simulink model "p7"  (R2020a)
settings: Solver=VariableStepAuto  StartTime=0.0  StopTime=10.0  RelTol=1e-3
model workspace (MAT data in the model file):
  A = Simulink.Parameter
  A.Value = 1
  A.DataType = 'auto'
  A.Dimensions = [1 1]
  B = Simulink.Parameter
  B.Value = 2
  B.DataType = 'auto'
  B.Dimensions = [1 1]
  C = Simulink.Parameter
  C.Value = -1
  C.DataType = 'auto'
  C.Dimensions = [1 1]
  D = Simulink.Parameter
  D.Value = 1
  D.DataType = 'auto'
  D.Dimensions = [1 1]
  E = Simulink.Parameter
  E.Value = 1
  E.DataType = 'auto'
  E.Dimensions = [1 1]
  F = Simulink.Parameter
  F.Value = -1
  F.DataType = 'auto'
  F.Dimensions = [1 1]
settings Model: Creator=007  LastModifiedBy=007

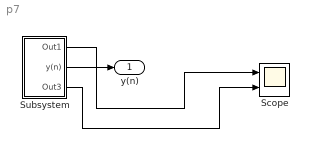
== system p7 ==
  Scope : Scope  NumInputPorts=2
  Subsystem : Subsystem
  y(n) : Outport
  wires:
  Subsystem/1(Out1) -> Scope/1
  Subsystem/2(y(n)) -> y(n)/1
  Subsystem/3(Out3) -> Scope/2

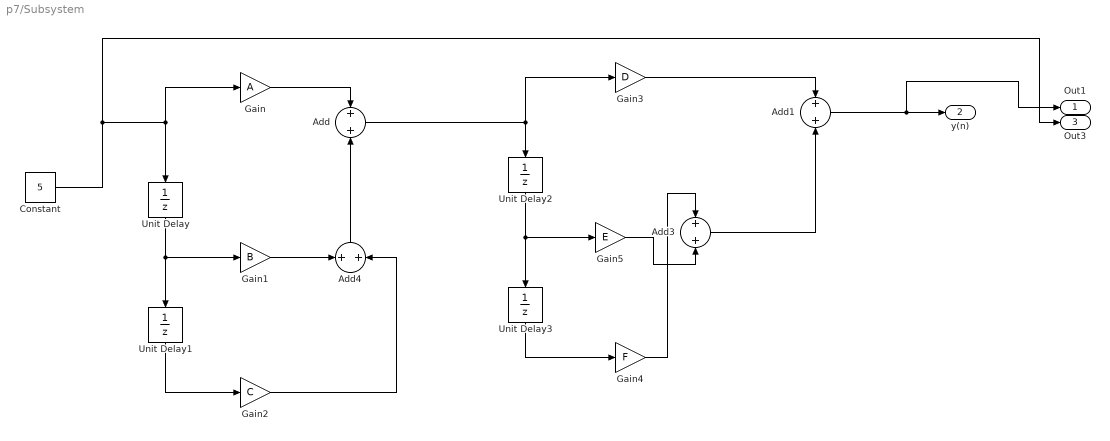
== system p7/Subsystem ==
  Add{,1,3..4} (4 alike) : Sum
  Constant : Constant  Value=5
  Gain : Gain  Gain=A
  Gain1 : Gain  Gain=B
  Gain2 : Gain  Gain=C
  Gain3 : Gain  Gain=D
  Gain4 : Gain  Gain=F
  Gain5 : Gain  Gain=E
  Unit Delay{,1..3} (4 alike) : UnitDelay  SampleTime=-1  HasFrameUpgradeWarning=on
  Out1 : Outport
  y(n) : Outport  Port=2
  Out3 : Outport  Port=3
  wires:
  Add/1 -> Unit Delay2/1, Gain3/1
  Gain/1 -> Add/1
  Gain5/1 -> Add3/2
  Unit Delay2/1 -> Unit Delay3/1, Gain5/1
  Add4/1 -> Add/2
  Add3/1 -> Add1/2
  Unit Delay1/1 -> Gain2/1
  Add1/1 -> y(n)/1, Out1/1
  Gain4/1 -> Add3/1
  Constant/1 -> Out3/1, Unit Delay/1, Gain/1
  Unit Delay3/1 -> Gain4/1
  Unit Delay/1 -> Unit Delay1/1, Gain1/1
  Gain1/1 -> Add4/1
  Gain3/1 -> Add1/1
  Gain2/1 -> Add4/2
